simulink subsystem "controller"  (R2020b)
settings: Solver=VariableStepAuto  StartTime=0.0  StopTime=10.0  RelTol=1e-3
undefined symbols (not defined in the file): T_c
settings Model: Creator=leop9  LastModifiedBy=Lenyor

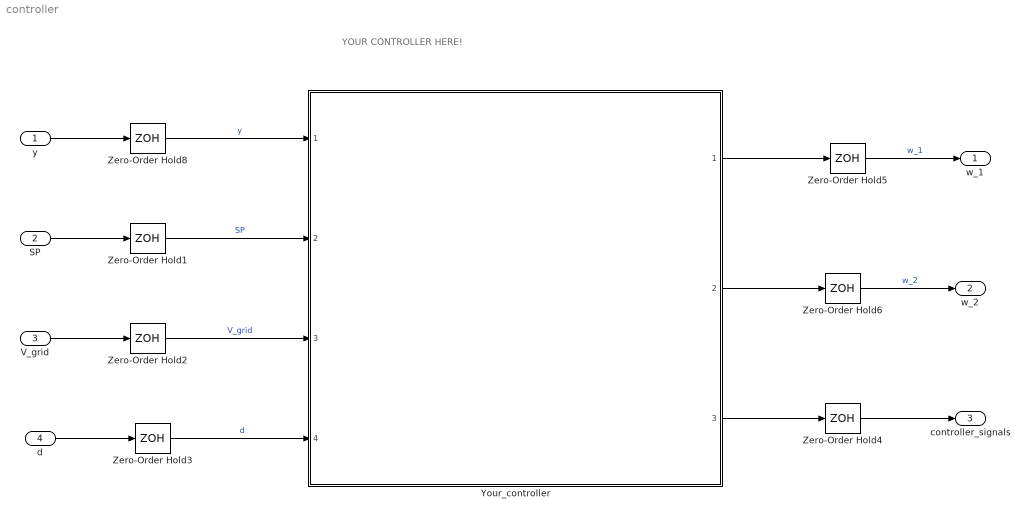
== system controller ==
  note: YOUR CONTROLLER HERE!
  y : Inport
  SP : Inport  Port=2
  V_grid : Inport  Port=3
  d : Inport  Port=4
  Your_controller : Subsystem  ReferencedSubsystem=PI_original
  Zero-Order Hold{1..6,8} (7 alike) : ZeroOrderHold  SampleTime=T_c
  w_1 : Outport
  w_2 : Outport  Port=2
  controller_signals : Outport  Port=3
  wires:
  Zero-Order Hold5/1 -> w_1/1  "w_1"
  Zero-Order Hold6/1 -> w_2/1  "w_2"
  y/1 -> Zero-Order Hold8/1
  SP/1 -> Zero-Order Hold1/1
  V_grid/1 -> Zero-Order Hold2/1
  d/1 -> Zero-Order Hold3/1
  Your_controller/1 -> Zero-Order Hold5/1
  Your_controller/2 -> Zero-Order Hold6/1
  Zero-Order Hold4/1 -> controller_signals/1
  Your_controller/3 -> Zero-Order Hold4/1
  Zero-Order Hold8/1 -> Your_controller/1  "y"
  Zero-Order Hold3/1 -> Your_controller/4  "d"
  Zero-Order Hold2/1 -> Your_controller/3  "V_grid"
  Zero-Order Hold1/1 -> Your_controller/2  "SP"
